simulink model "Fibonacci_number"  (R2019b)
settings: Solver=FixedStepAuto  StartTime=0.0  StopTime=5  FixedStep=1  RelTol=1e-3
settings Model: Creator=Rashedul Islam  LastModifiedBy=Rashedul Islam

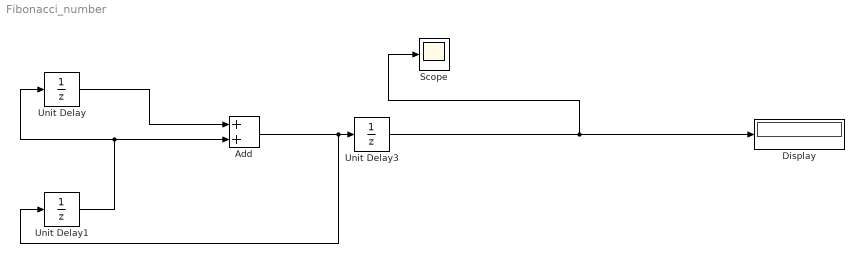
== system Fibonacci_number ==
  Add : Sum
  Display : Display
  Scope : Scope
  Unit Delay : UnitDelay  SampleTime=-1  HasFrameUpgradeWarning=on
  Unit Delay1 : UnitDelay  InitialCondition=1  SampleTime=-1  HasFrameUpgradeWarning=on
  Unit Delay3 : UnitDelay  SampleTime=-1  HasFrameUpgradeWarning=on
  wires:
  Unit Delay/1 -> Add/1
  Unit Delay1/1 -> Unit Delay/1, Add/2
  Add/1 -> Unit Delay3/1, Unit Delay1/1
  Unit Delay3/1 -> Scope/1, Display/1
